simulink model "Homework1"  (R2024a)
settings: Solver=VariableStepAuto  StartTime=0.0  StopTime=10.0  RelTol=1e-3
undefined symbols (not defined in the file): Iarated, Ifrated, J, k0, k1, k2, k3, kf, ki_a, ki_w, kp_a, kp_w, La, Ra, vrated, wref
libraries: slpidlib x2
settings Model: Creator=natha  LastModifiedBy=natha

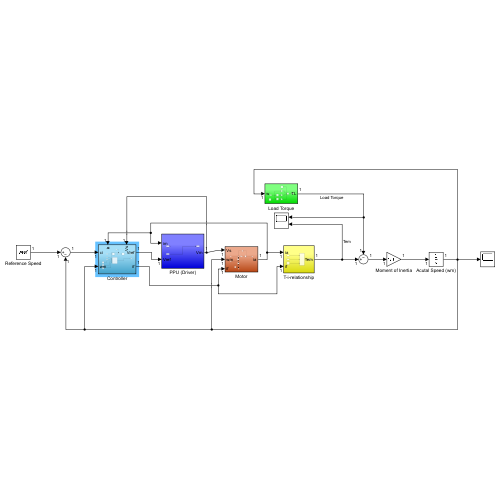
[thumbnail: Simulink's stored preview of the top-level diagram]
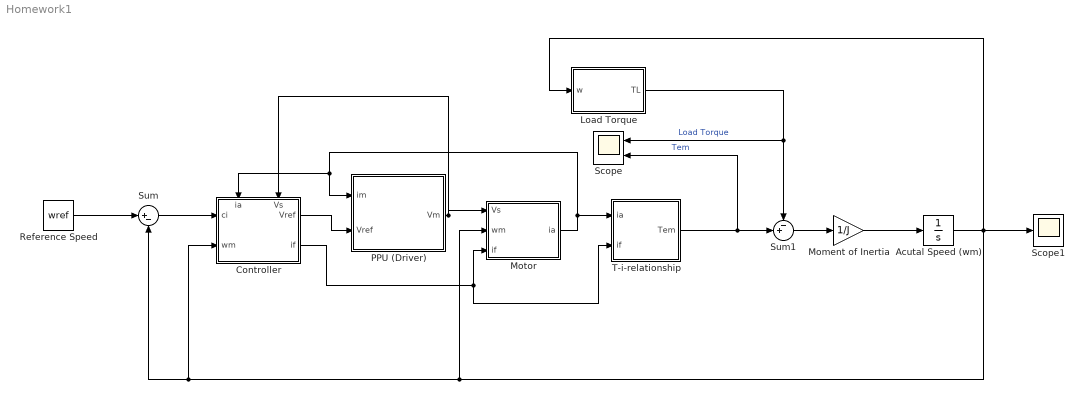
== system Homework1 ==
  Acutal Speed (wm) : Integrator
  Controller : Subsystem
      settings: PortSchema="{\"entries\":[{\"content\":{\"sides\":[{\"content\":{\"connectorIds\":[\"In1\",\"In2\"]},\"type\":\"ConnectorPlacement.EquallySpacedRectSide\",\"uuid\":\"bb364eb7-fe2e-4b30-a416-00f7c1cb992e\"},{\"content\":{\"connectorIds\":[\"Out1\",\"Out2\"],\"side\":\"RIGHT\"},\"type\":\"ConnectorPlacement.EquallySpacedRectSide\",\"uuid\":\"4bbb6234-647d-4276-b828-5a6565b9e037\"},{\"content\":{\"connectorIds\":[\"In3\",\"In4\"],\"side\":\"TOP\"},\"type\":\"ConnectorPlacement.EquallySpacedRectSide\",\"uuid\":\"2651ecb8-1b6d-48db-b083-649fd9f84285\"}]},\"type\":\"ConnectorPlacement.EquallySpacedConnector\",\"uuid\":\"5e05b9a4-eee3-4252-bfa8-b9c4d29fe4ea\"}],\"packageUris\":[\"http://schema.mathworks.com/mf0/Connector/R2020b\"],\"version\":\"1.0\"}"
  Load Torque : Subsystem
  Moment of Inertia : Gain  Gain=1/J
  Motor : Subsystem
  PPU (Driver) : Subsystem
  Reference Speed : Constant  Value=wref
  Scope : Scope  NumInputPorts=2
  Scope1 : Scope
  Sum : Sum  Inputs=|+-
  Sum1 : Sum  Inputs=-+|
  T-i-relationship : Subsystem
  wires:
  Reference Speed/1 -> Sum/1
  Acutal Speed (wm)/1 -> Motor/2(wm), Controller/2(wm), Sum/2, Scope1/1, Load Torque/1(w)
  Sum/1 -> Controller/1(ci)
  Controller/1(Vref) -> PPU (Driver)/2(Vref)
  PPU (Driver)/1(Vm) -> Controller/4(Vs), Motor/1(Vs)
  Motor/1(ia) -> T-i-relationship/1(ia), Controller/3(ia), PPU (Driver)/1(im)
  T-i-relationship/1(Tem) -> Sum1/2, Scope/2  "Tem"
  Load Torque/1(TL) -> Sum1/1, Scope/1  "Load Torque"
  Sum1/1 -> Moment of Inertia/1
  Moment of Inertia/1 -> Acutal Speed (wm)/1
  Controller/2(if) -> T-i-relationship/2(if), Motor/3(if)

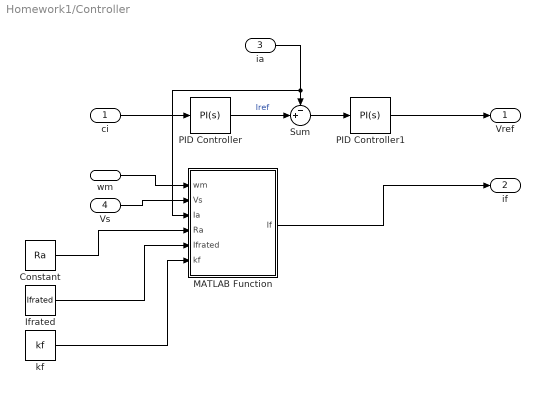
== system Homework1/Controller ==
  ci : Inport
  wm : Inport  Port=2
  ia : Inport  Port=3
  Vs : Inport  Port=4
  Constant : Constant  Value=Ra
  Ifrated : Constant  Value=Ifrated
  MATLAB Function : MATLAB Function  TreatAsAtomicUnit=on
  PID Controller : slpidlib/PID Controller  Controller=PI  Form=Parallel  TimeDomain=Continuous-time  UseExternalTs=off  SampleTime=-1  IntegratorMethod=Forward Euler  FilterMethod=Forward Euler  ControllerParametersSource=internal  P=kp_w  I=ki_w  UseKiTs=off  D=0  UseExternalDerivativeSource=off  N=100  UseFilter=on  TunerSelectOption=Transfer Function Based (PID Tuner App)  InitialConditionSource=internal  InitialConditionForIntegrator=0  InitialConditionForFilter=0  DifferentiatorICPrevScaledInput=0  ExternalReset=none  TrackingMode=off  Kt=1  LimitOutput=on  SatLimitsSource=internal  UpperSaturationLimit=Iarated  LowerSaturationLimit=-Iarated  LinearizeAsGain=on  AntiWindupMode=none  Kb=1  LimitIntegrator=off  UpperIntegratorSaturationLimit=inf  LowerIntegratorSaturationLimit=-inf  POutMin=[]  POutMax=[]  IOutMin=[]  IOutMax=[]  DOutMin=[]  DOutMax=[]  NOutMin=[]  NOutMax=[]  SumOutMin=[]  SumOutMax=[]  SaturationOutMin=[]  SaturationOutMax=[]  PParamMin=[]  PParamMax=[]  IParamMin=[]  IParamMax=[]  DParamMin=[]  DParamMax=[]  NParamMin=[]  NParamMax=[]  KbParamMin=[]  KbParamMax=[]  KtParamMin=[]  KtParamMax=[]  KbOutMin=[]  KbOutMax=[]  KtOutMin=[]  KtOutMax=[]  IntegratorOutMin=[]  IntegratorOutMax=[]  FilterOutMin=[]  FilterOutMax=[]  SumI1OutMin=[]  SumI1OutMax=[]  SumI2OutMin=[]  SumI2OutMax=[]  SumI3OutMin=[]  SumI3OutMax=[]  SumI4OutMin=[]  SumI4OutMax=[]  SumDOutMin=[]  SumDOutMax=[]  DifferentiatorOutMin=[]  DifferentiatorOutMax=[]  FilterDiffOutCoefMin=[]  FilterDiffOutCoefMax=[]  ReciprocalOutMin=[]  ReciprocalOutMax=[]  SumDenOutMin=[]  SumDenOutMax=[]  SumNumOutMin=[]  SumNumOutMax=[]  DivideOutMin=[]  DivideOutMax=[]  UdiffTsProdOutMin=[]  UdiffTsProdOutMax=[]  NTsProdOutMin=[]  NTsProdOutMax=[]  UintegralTsProdOutMin=[]  UintegralTsProdOutMax=[]  UngainTsProdOutMin=[]  UngainTsProdOutMax=[]  ClampingZeroOutDataTypeStr=Inherit: Inherit via back propagation  ClampingZeroOutMin=[]  ClampingZeroOutMax=[]  FilterDenConstantOutDataTypeStr=Inherit: Inherit via back propagation  FilterDenConstantOutMin=[]  FilterDenConstantOutMax=[]  PCopyOutDataTypeStr=Inherit: Inherit via back propagation  PCopyOutMin=[]  PCopyOutMax=[]  NCopyOutDataTypeStr=Inherit: Inherit via back propagation  NCopyOutMin=[]  NCopyOutMax=[]  IntegratorContinuousStateAttributes=''  IntegratorStateMustResolveToSignalObject=off  IntegratorRTWStateStorageClass=Auto  FilterContinuousStateAttributes=''  FilterStateMustResolveToSignalObject=off  FilterRTWStateStorageClass=Auto  ParallelPVariant=InternalParameters  IdealPVariant=Disabled  IVariant=InternalParameters  DVariant=Disabled  IntegratorVariant=Continuous  SatVariant=Enabled  AWVariant=Passthrough  PCopyVariant=Disabled  TRVariant=Disabled  FdbkBlocksVariant=Forward  IdealPFdbkVariant=Disabled  SatFdbkVariant=Disabled  DerivativeFilterVariant=Disabled  NVariant=Disabled  NCopyVariant=Disabled_SignalSpec  FilterICVariant=Disabled  IntegratorICVariant=InternalICs  ExternalResetVariant=Disabled  TRSumVariant=Passthrough  SumFdbkVariant=Disabled  SumVariant=Sum_PI  TsampFilterVariant=InternalTs  TsampNgainVariant=Passthrough  TsampIntegralVariant=Disabled_SignalSpec  ExternalSaturationOutDataTypeStr=Inherit: Same as second input  DerivativeSourceVariant=Disabled
  PID Controller1 : slpidlib/PID Controller  Controller=PI  Form=Parallel  TimeDomain=Continuous-time  UseExternalTs=off  SampleTime=-1  IntegratorMethod=Forward Euler  FilterMethod=Forward Euler  ControllerParametersSource=internal  P=kp_a  I=ki_a  UseKiTs=off  D=0  UseExternalDerivativeSource=off  N=100  UseFilter=on  TunerSelectOption=Transfer Function Based (PID Tuner App)  InitialConditionSource=internal  InitialConditionForIntegrator=0  InitialConditionForFilter=0  DifferentiatorICPrevScaledInput=0  ExternalReset=none  TrackingMode=off  Kt=1  LimitOutput=on  SatLimitsSource=internal  UpperSaturationLimit=vrated  LowerSaturationLimit=-vrated  LinearizeAsGain=on  AntiWindupMode=none  Kb=1  LimitIntegrator=off  UpperIntegratorSaturationLimit=inf  LowerIntegratorSaturationLimit=-inf  POutMin=[]  POutMax=[]  IOutMin=[]  IOutMax=[]  DOutMin=[]  DOutMax=[]  NOutMin=[]  NOutMax=[]  SumOutMin=[]  SumOutMax=[]  SaturationOutMin=[]  SaturationOutMax=[]  PParamMin=[]  PParamMax=[]  IParamMin=[]  IParamMax=[]  DParamMin=[]  DParamMax=[]  NParamMin=[]  NParamMax=[]  KbParamMin=[]  KbParamMax=[]  KtParamMin=[]  KtParamMax=[]  KbOutMin=[]  KbOutMax=[]  KtOutMin=[]  KtOutMax=[]  IntegratorOutMin=[]  IntegratorOutMax=[]  FilterOutMin=[]  FilterOutMax=[]  SumI1OutMin=[]  SumI1OutMax=[]  SumI2OutMin=[]  SumI2OutMax=[]  SumI3OutMin=[]  SumI3OutMax=[]  SumI4OutMin=[]  SumI4OutMax=[]  SumDOutMin=[]  SumDOutMax=[]  DifferentiatorOutMin=[]  DifferentiatorOutMax=[]  FilterDiffOutCoefMin=[]  FilterDiffOutCoefMax=[]  ReciprocalOutMin=[]  ReciprocalOutMax=[]  SumDenOutMin=[]  SumDenOutMax=[]  SumNumOutMin=[]  SumNumOutMax=[]  DivideOutMin=[]  DivideOutMax=[]  UdiffTsProdOutMin=[]  UdiffTsProdOutMax=[]  NTsProdOutMin=[]  NTsProdOutMax=[]  UintegralTsProdOutMin=[]  UintegralTsProdOutMax=[]  UngainTsProdOutMin=[]  UngainTsProdOutMax=[]  ClampingZeroOutDataTypeStr=Inherit: Inherit via back propagation  ClampingZeroOutMin=[]  ClampingZeroOutMax=[]  FilterDenConstantOutDataTypeStr=Inherit: Inherit via back propagation  FilterDenConstantOutMin=[]  FilterDenConstantOutMax=[]  PCopyOutDataTypeStr=Inherit: Inherit via back propagation  PCopyOutMin=[]  PCopyOutMax=[]  NCopyOutDataTypeStr=Inherit: Inherit via back propagation  NCopyOutMin=[]  NCopyOutMax=[]  IntegratorContinuousStateAttributes=''  IntegratorStateMustResolveToSignalObject=off  IntegratorRTWStateStorageClass=Auto  FilterContinuousStateAttributes=''  FilterStateMustResolveToSignalObject=off  FilterRTWStateStorageClass=Auto  ParallelPVariant=InternalParameters  IdealPVariant=Disabled  IVariant=InternalParameters  DVariant=Disabled  IntegratorVariant=Continuous  SatVariant=Enabled  AWVariant=Passthrough  PCopyVariant=Disabled  TRVariant=Disabled  FdbkBlocksVariant=Forward  IdealPFdbkVariant=Disabled  SatFdbkVariant=Disabled  DerivativeFilterVariant=Disabled  NVariant=Disabled  NCopyVariant=Disabled_SignalSpec  FilterICVariant=Disabled  IntegratorICVariant=InternalICs  ExternalResetVariant=Disabled  TRSumVariant=Passthrough  SumFdbkVariant=Disabled  SumVariant=Sum_PI  TsampFilterVariant=InternalTs  TsampNgainVariant=Passthrough  TsampIntegralVariant=Disabled_SignalSpec  ExternalSaturationOutDataTypeStr=Inherit: Same as second input  DerivativeSourceVariant=Disabled
  Sum : Sum  Inputs=-+|
  kf : Constant  Value=kf
  Vref : Outport
  if : Outport  Port=2
  wires:
  ci/1 -> PID Controller/1
  PID Controller/1 -> Sum/2  "Iref"
  ia/1 -> MATLAB Function/3(Ia), Sum/1
  Sum/1 -> PID Controller1/1
  PID Controller1/1 -> Vref/1
  wm/1 -> MATLAB Function/1(wm)
  Vs/1 -> MATLAB Function/2(Vs)
  Constant/1 -> MATLAB Function/4(Ra)
  MATLAB Function/1(If) -> if/1
  Ifrated/1 -> MATLAB Function/5(Ifrated)
  kf/1 -> MATLAB Function/6(kf)

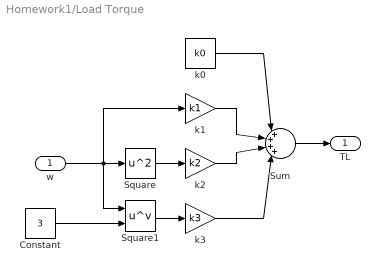
== system Homework1/Load Torque ==
  w : Inport
  Constant : Constant  Value=3
  Square : Math  Operator=square
  Square1 : Math  Operator=pow
  Sum : Sum  Inputs=|++++|
  k0 : Constant  Value=k0
  k1 : Gain  Gain=k1
  k2 : Gain  Gain=k2
  k3 : Gain  Gain=k3
  TL : Outport
  wires:
  w/1 -> Square/1, Square1/1, k1/1
  Square/1 -> k2/1
  Constant/1 -> Square1/2
  Square1/1 -> k3/1
  k0/1 -> Sum/1
  k1/1 -> Sum/2
  k2/1 -> Sum/3
  k3/1 -> Sum/4
  Sum/1 -> TL/1

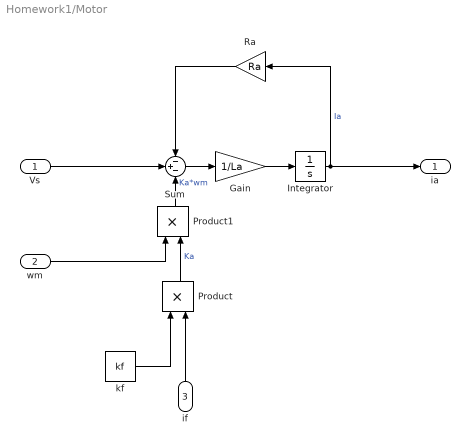
== system Homework1/Motor ==
  Vs : Inport
  wm : Inport  Port=2
  if : Inport  Port=3
  Gain : Gain  Gain=1/La
  Integrator : Integrator
  Product : Product
  Product1 : Product
  Ra : Gain  Gain=Ra
  Sum : Sum  Inputs=-+-
  kf : Constant  Value=kf
  ia : Outport
  wires:
  Integrator/1 -> Ra/1, ia/1  "Ia"
  Gain/1 -> Integrator/1
  Sum/1 -> Gain/1
  Ra/1 -> Sum/1
  Vs/1 -> Sum/2
  if/1 -> Product/2
  kf/1 -> Product/1
  Product1/1 -> Sum/3  "Ka*wm"
  wm/1 -> Product1/1
  Product/1 -> Product1/2  "Ka"

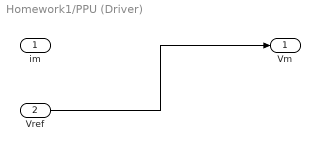
== system Homework1/PPU (Driver) ==
  im : Inport
  Vref : Inport  Port=2
  Vm : Outport
  wires:
  Vref/1 -> Vm/1

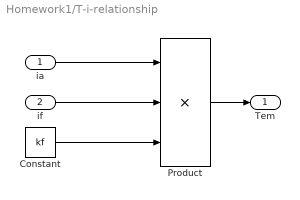
== system Homework1/T-i-relationship ==
  ia : Inport
  if : Inport  Port=2
  Constant : Constant  Value=kf
  Product : Product  Inputs=3
  Tem : Outport
  wires:
  Constant/1 -> Product/3
  ia/1 -> Product/1
  if/1 -> Product/2
  Product/1 -> Tem/1

== matlab function Homework1/Controller/MATLAB Function ==
  data: wm input; If output; Vs input; Ia input; Ra input; Ifrated input; kf input
function If = fcn(wm, Vs, Ia, Ra, Ifrated, kf)

If = (Vs - Ia * Ra) / (kf * wm);
if abs(If) > Ifrated
    If = Ifrated;
end
